simulink model "RLC"  (R2019a)
settings: Solver=VariableStepAuto  StartTime=0.0  StopTime=10.0  RelTol=1e-3
values from neighbouring files (symbols this model uses):
  C = 1    [value.m]
  L = 1    [value.m]
  R = 1    [value.m]
settings Model: Creator=Takumi SHIOTA  LastModifiedBy=Takumi SHIOTA

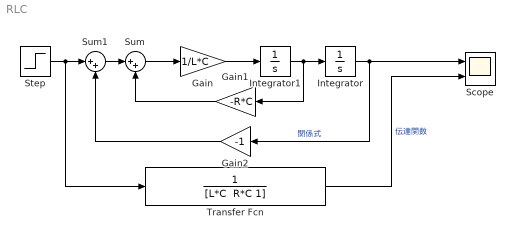
== system RLC ==
  Gain : Gain  Gain=1/L*C
  Gain1 : Gain  Gain=-R*C
  Gain2 : Gain  Gain=-1
  Integrator : Integrator
  Integrator1 : Integrator
  Scope : Scope  NumInputPorts=2
  Step : Step  SampleTime=0
  Sum : Sum  Inputs=|++
  Sum1 : Sum  Inputs=|++
  Transfer Fcn : TransferFcn  Denominator="[L*C  R*C 1]"
  wires:
  Gain1/1 -> Sum/2
  Transfer Fcn/1 -> Scope/2  "伝達関数"
  Gain/1 -> Integrator1/1
  Step/1 -> Sum1/1, Transfer Fcn/1
  Sum/1 -> Gain/1
  Integrator/1 -> Gain2/1, Scope/1  "関係式"
  Sum1/1 -> Sum/1
  Gain2/1 -> Sum1/2
  Integrator1/1 -> Gain1/1, Integrator/1
